simulink model "vector_gain"  (R2020b)
settings: Solver=FixedStepDiscrete  StartTime=0.0  StopTime=stopTime  RelTol=1e-3
InitFcn:
  | initCallback
StopFcn:
  | stopCallback
model workspace (MAT data in the model file):
  HDLVAXIMasterConfig = hdlverifier.internal.AXIMaster.ConfigParams
  HDLVAXIMasterConfig.Vendor = 'Intel'
  HDLVAXIMasterConfig.JTAGWasConfigured = 1
undefined symbols (not defined in the file or in its folder): config
settings Model: SimulationMode=accelerator  Creator=Ross  LastModifiedBy=wickh
settings SolverCC: AutoInsertRateTranBlk=on
settings DataIOCC: ReturnWorkspaceOutputs=off
settings OptimizationCC: BlockReduction=off  ConditionallyExecuteInputs=off  DefaultParameterBehavior=Inlined
settings DebuggingCC: SignalInfNanChecking=error  SignalRangeChecking=warning  ReadBeforeWriteMsg=DisableAll  WriteAfterWriteMsg=DisableAll  WriteAfterReadMsg=DisableAll  AlgebraicLoopMsg=error  MultiTaskDSMMsg=none  SingleTaskRateTransMsg=error  ParameterUnderflowMsg=warning  UnderSpecifiedDataTypeMsg=error  PregeneratedLibrarySubsystemCodeDiagnostic=none  ArithmeticOperatorsInVariantConditions=warning
settings HardwareCC: ProdBitPerPointer=32  ProdBitPerSizeT=32  ProdBitPerPtrDiffT=32  ProdLargestAtomicFloat=None  ProdIntDivRoundTo=Undefined  ProdEndianess=Unspecified  ProdWordSize=32  ProdHWDeviceType=ASIC/FPGA->ASIC/FPGA  TargetBitPerPointer=64  TargetBitPerSizeT=64  TargetBitPerPtrDiffT=64  TargetLongLongMode=on  TargetIntDivRoundTo=Zero  TargetEndianess=LittleEndian  TargetWordSize=64  TargetHWDeviceType=Custom Processor->MATLAB Host Computer  ProdEqTarget=off
settings ModelReferenceCC: UpdateModelReferenceTargets=IfOutOfDate
settings SFSimCC: SFSimEcho=off  SimUseLocalCustomCode=off  CustomCodeUndefinedFunction=UseInterfaceOnly
settings RTWCC: RTWUseLocalCustomCode=off

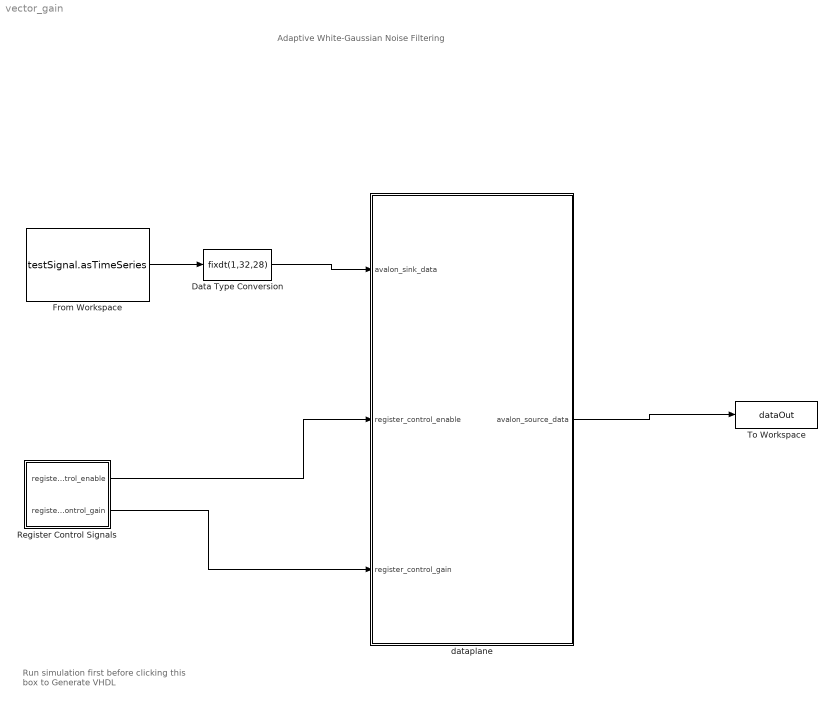
== system vector_gain ==
  note: Adaptive White-Gaussian Noise Filtering
  note: Run simulation first
      | before clicking this box to
      | Generate VHDL
  Data Type Conversion : DataTypeConversion  OutDataTypeStr=fixdt(1,32,28)
  From Workspace : FromWorkspace  VariableName=testSignal.asTimeSeries  OutDataTypeStr=double  SampleTime=1 / config.system.sampleClockFrequency  Interpolate=off  OutputAfterFinalValue=Setting to zero
  Register Control Signals : Subsystem
  To Workspace : ToWorkspace  VariableName=dataOut  SaveFormat=Timeseries  SampleTime=-1
      settings: Save2DSignal=2-D array (concatenate along first dimension)
  dataplane : Subsystem  TreatAsAtomicUnit=on
  wires:
  dataplane/1(avalon_source_data) -> To Workspace/1
  From Workspace/1 -> Data Type Conversion/1
  Data Type Conversion/1 -> dataplane/1(avalon_sink_data)
  Register Control Signals/1(register_control_enable) -> dataplane/2(register_control_enable)
  Register Control Signals/2(register_control_gain) -> dataplane/3(register_control_gain)

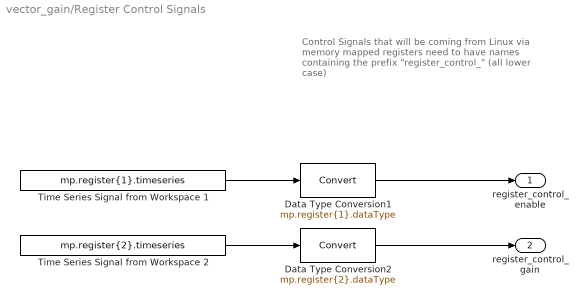
== system vector_gain/Register Control Signals ==
  note: Control Signals that will be coming from Linux via
      | memory mapped registers need to have names
      | containing the prefix "register_control_"
      | (all lower case)
  Data Type Conversion1 : DataTypeConversion  OutDataTypeStr=mp.register{1}.dataType
  Data Type Conversion2 : DataTypeConversion  OutDataTypeStr=mp.register{2}.dataType
  Time Series Signal from Workspace 1 : FromWorkspace  VariableName=mp.register{1}.timeseries  OutDataTypeStr=double  SampleTime=1 / config.system.sampleClockFrequency
  Time Series Signal from Workspace 2 : FromWorkspace  VariableName=mp.register{2}.timeseries  OutDataTypeStr=double  SampleTime=1 / config.system.sampleClockFrequency
  register_control_enable : Outport  VectorParamsAs1DForOutWhenUnconnected=off
  register_control_gain : Outport  Port=2  VectorParamsAs1DForOutWhenUnconnected=off
  wires:
  Time Series Signal from Workspace 1/1 -> Data Type Conversion1/1
  Data Type Conversion1/1 -> register_control_enable/1
  Time Series Signal from Workspace 2/1 -> Data Type Conversion2/1
  Data Type Conversion2/1 -> register_control_gain/1

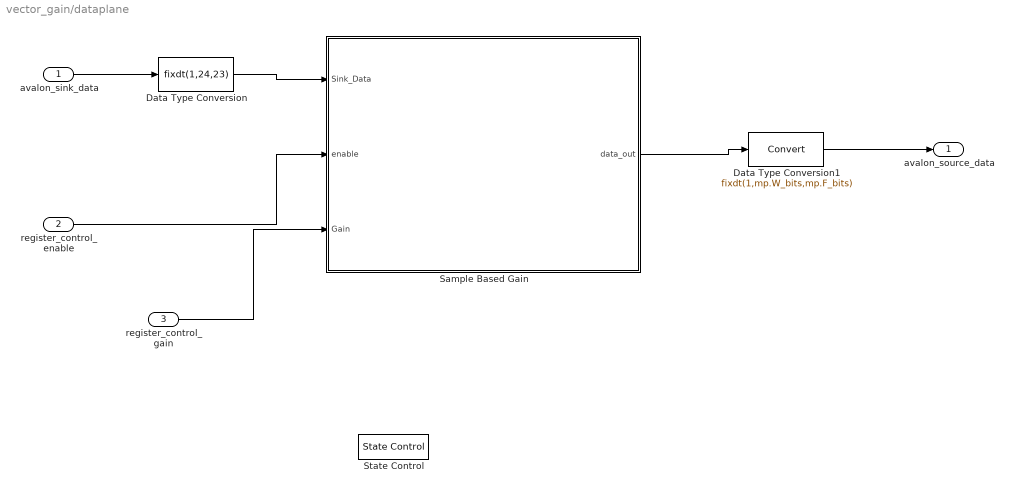
== system vector_gain/dataplane ==
  avalon_sink_data : Inport
  register_control_enable : Inport  Port=2
  register_control_gain : Inport  Port=3
  Data Type Conversion : DataTypeConversion  OutDataTypeStr=fixdt(1,24,23)
  Data Type Conversion1 : DataTypeConversion  OutDataTypeStr=fixdt(1,mp.W_bits,mp.F_bits)
  Sample Based Gain : Subsystem
  State Control : StateControl  StateControl=Synchronous
  avalon_source_data : Outport  VectorParamsAs1DForOutWhenUnconnected=off
  wires:
  Data Type Conversion1/1 -> avalon_source_data/1
  avalon_sink_data/1 -> Data Type Conversion/1
  register_control_enable/1 -> Sample Based Gain/2(enable)
  Data Type Conversion/1 -> Sample Based Gain/1(Sink_Data)
  register_control_gain/1 -> Sample Based Gain/3(Gain)
  Sample Based Gain/1(data_out) -> Data Type Conversion1/1

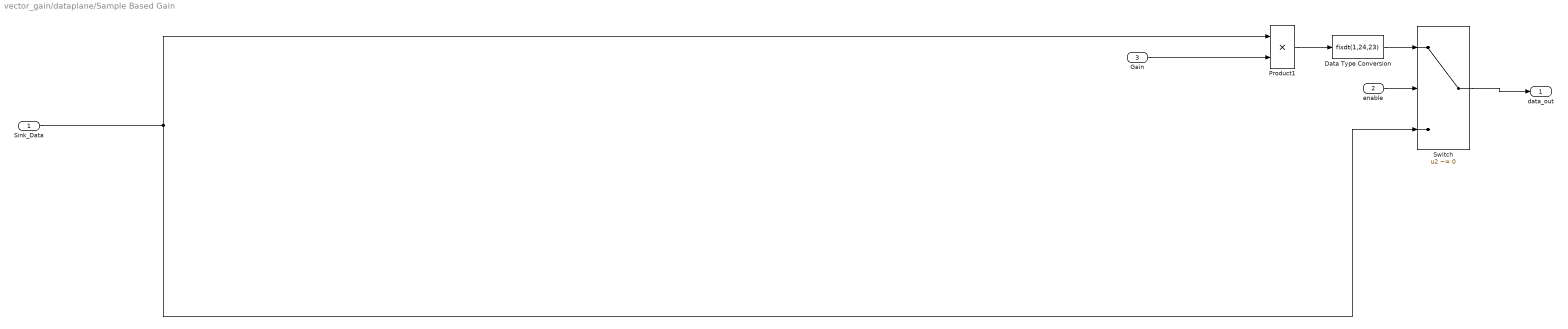
== system vector_gain/dataplane/Sample Based Gain ==
  Sink_Data : Inport
  enable : Inport  Port=2
  Gain : Inport  Port=3
  Data Type Conversion : DataTypeConversion  OutDataTypeStr=fixdt(1,24,23)
  Product1 : Product
  Switch : Switch  Criteria=u2 ~= 0
  data_out : Outport
  wires:
  Sink_Data/1 -> Product1/1, Switch/3
  Product1/1 -> Data Type Conversion/1
  Switch/1 -> data_out/1
  enable/1 -> Switch/2
  Gain/1 -> Product1/2
  Data Type Conversion/1 -> Switch/1
